simulink model "quartercar"  (R2015b)
settings: Solver=ode15s  StartTime=0  StopTime=5  RelTol=1e-4
model workspace (MAT data in the model file):
  K_d = 230717.117936
  K_i = 343500690.022
  K_p = 458682142.598
  b = 350
  b1 = 350
  b2 = 15020
  k1 = 80000
  k2 = 500000
  m1 = 2500
  m2 = 320
  road_step = -1
settings Model: Creator=jyotirmoy  LastModifiedBy=xjin
settings DataIOCC: LimitDataPoints=off  SaveFormat=Structure  SaveState=on  StateSaveName=xoutNew  OutputSaveName=youtNew  OutputOption=AdditionalOutputTimes  OutputTimes=[0,0.1,0.2,0.3,0.4,0.5,0.6,0.7,0.8,0.9,1,1.1,1.2,1.3,1.4,1.5,1.6,1.7,1.8,1.9,2,2.1,2.2,2.3,2.4,2.5,2.6,2.7,2.8,2.9,3,3.1,3.2,3.3,3.4,3.5,3.6,3.7,3.8,3.9,4,4.1,4.2,4.3,4.4,4.5,4.6,4.7,4.8,4.9,5]
settings DebuggingCC: UnderspecifiedInitializationDetection=Classic  MergeDetectMultiDrivingBlocksExec=none  SolverPrmCheckMsg=warning  StateNameClashWarn=warning
settings HardwareCC: ProdBitPerPointer=32  ProdLargestAtomicFloat=None  ProdIntDivRoundTo=Undefined  ProdEndianess=Unspecified  ProdWordSize=32  ProdHWDeviceType=32-bit Generic
settings GRTTargetCC: GeneratePreprocessorConditionals=Disable all
settings ConfigComp: CovModelRefEnable=Off

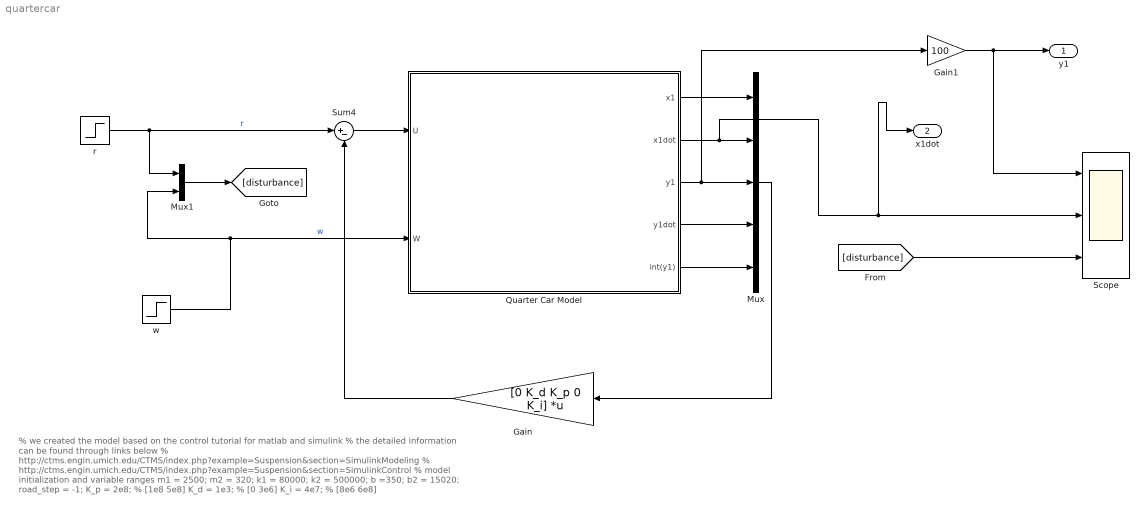
== system quartercar ==
  note: % we created the model based on the control tutorial for matlab and simulink
      | % the detailed information can be found through links below
      | % http://ctms.engin.umich.edu/CTMS/index.php?example=Suspension&section=SimulinkModeling
      | % http://ctms.engin.umich.edu/CTMS/index.php?example=Suspension&section=SimulinkControl
      | % model initialization and variable ranges
      |
      | m1 = 2500;
      | m2 = 320;
      | k1 = 80000;
      | k2 = 500000;
      | b =350;
      | b2 = 15020;
      | road_step = -1;
      | K_p = 2e8; % [1e8 5e8]
      | K_d = 1e3; % [0 3e6]
      | K_i = 4e7;  % [8e6 6e8]
  Gain : Gain  Gain=[0 K_d K_p 0 K_i]  Multiplication=Matrix(K*u)
  Gain1 : Gain  Gain=100
  Mux : Mux  Inputs=5
  Mux1 : Mux  Inputs=2
  Quarter Car Model : Subsystem
  Scope : Scope  NumInputPorts=3
  Sum4 : Sum  Inputs=|+-
  r : Step  After=0  SampleTime=0
  w : Step  Time=0  After=road_step  SampleTime=0
  y1 : Outport
  x1dot : Outport  Port=2
  wires:
  r/1 -> Sum4/1, Mux1/1  "r"
  Sum4/1 -> Quarter Car Model/1(U)
  w/1 -> Mux1/2, Quarter Car Model/2(W)  "w"
  Quarter Car Model/1(x1) -> Mux/1
  Quarter Car Model/3(y1) -> Gain1/1, Mux/3
  Quarter Car Model/4(y1dot) -> Mux/4
  Quarter Car Model/5(int(y1)) -> Mux/5
  Mux/1 -> Gain/1
  Gain/1 -> Sum4/2
  [disturbance] -> Scope/3
  Mux1/1 -> [disturbance]
  Quarter Car Model/2(x1dot) -> x1dot/1, Scope/2, Mux/2
  Gain1/1 -> Scope/1, y1/1

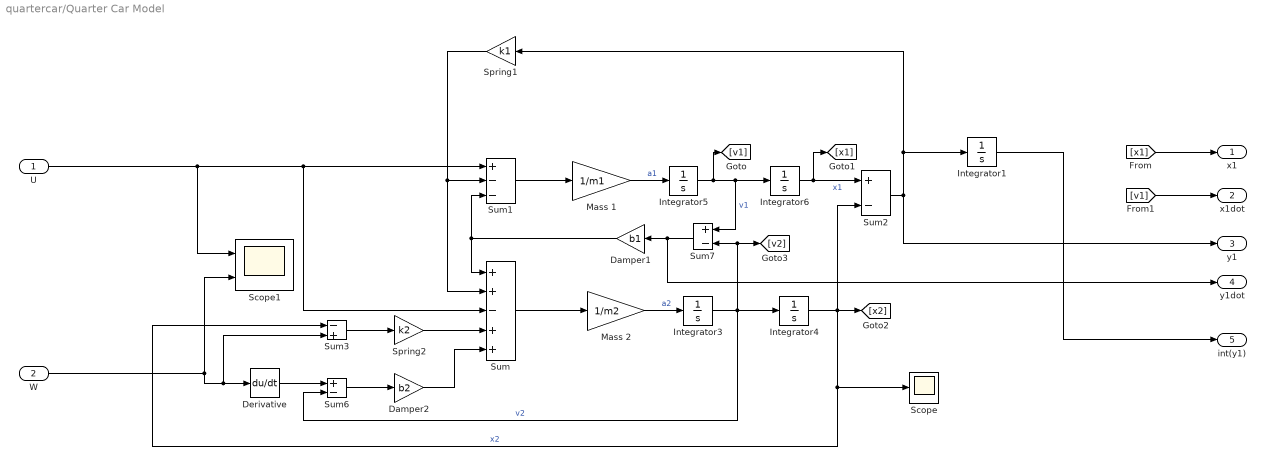
== system quartercar/Quarter Car Model ==
  U : Inport
  W : Inport  Port=2
  Damper1 : Gain  Gain=b1
  Damper2 : Gain  Gain=b2
  Derivative : Derivative
  Integrator{1,3..6} (5 alike) : Integrator
  Mass 1 : Gain  Gain=1/m1
  Mass 2 : Gain  Gain=1/m2
  Scope : Scope
  Scope1 : Scope  NumInputPorts=2
  Spring1 : Gain  Gain=k1
  Spring2 : Gain  Gain=k2
  Sum : Sum  Inputs=++-++
  Sum1 : Sum  Inputs=+--
  Sum2 : Sum  Inputs=+-
  Sum3 : Sum  Inputs=-+
  Sum6 : Sum  Inputs=+-
  Sum7 : Sum  Inputs=+-
  x1 : Outport
  x1dot : Outport  Port=2
  y1 : Outport  Port=3
  y1dot : Outport  Port=4
  int(y1) : Outport  Port=5
  wires:
  Mass 1/1 -> Integrator5/1  "a1"
  Integrator6/1 -> [x1], Sum2/1  "x1"
  Sum1/1 -> Mass 1/1
  Integrator5/1 -> [v1], Sum7/1, Integrator6/1  "v1"
  U/1 -> Scope1/1, Sum/3, Sum1/1
  Integrator4/1 -> Sum2/2, [x2], Scope/1, Sum3/1  "x2"
  Integrator3/1 -> Sum7/2, [v2], Sum6/2, Integrator4/1  "v2"
  Spring2/1 -> Sum/4
  Sum/1 -> Mass 2/1
  Sum7/1 -> y1dot/1, Damper1/1
  W/1 -> Sum3/2, Derivative/1, Scope1/2
  Sum2/1 -> Spring1/1, Integrator1/1, y1/1
  Spring1/1 -> Sum/2, Sum1/2
  Sum6/1 -> Damper2/1
  Damper1/1 -> Sum1/3, Sum/1
  Sum3/1 -> Spring2/1
  Mass 2/1 -> Integrator3/1  "a2"
  Damper2/1 -> Sum/5
  Derivative/1 -> Sum6/1
  [x1] -> x1/1
  [v1] -> x1dot/1
  Integrator1/1 -> int(y1)/1
